simulink model "OMAP_ver_MIL10"  (R2018b)
settings: Solver=FixedStepDiscrete  StartTime=0.0  StopTime=10.0  FixedStep=0.01  RelTol=1e-3
undefined symbols (not defined in the file or in its folder): OMAP_Switch_EMS, OMAP_Switch_EPS, OMAP_Switch_ESC, OMAP_Switch_IC, OMAP_Switch_OTHER, TH_HMIClb_tiDgrdIconWarnHiDurT_C, TH_HMIClb_tiDgrdIconWarnLoDurT_C, TH_HMIClb_tiDgrdVocWarnDurT_C, TH_HMIClb_tiHndOffTxtWarnT_C, TH_HMIClb_tiHndOffVocWarnT_C, TH_HMIClb_tiSWALimFlgDetT_C, TH_HMIClb_tiTxtLimT_C
libraries: simulink x118
(part 3 of 9)

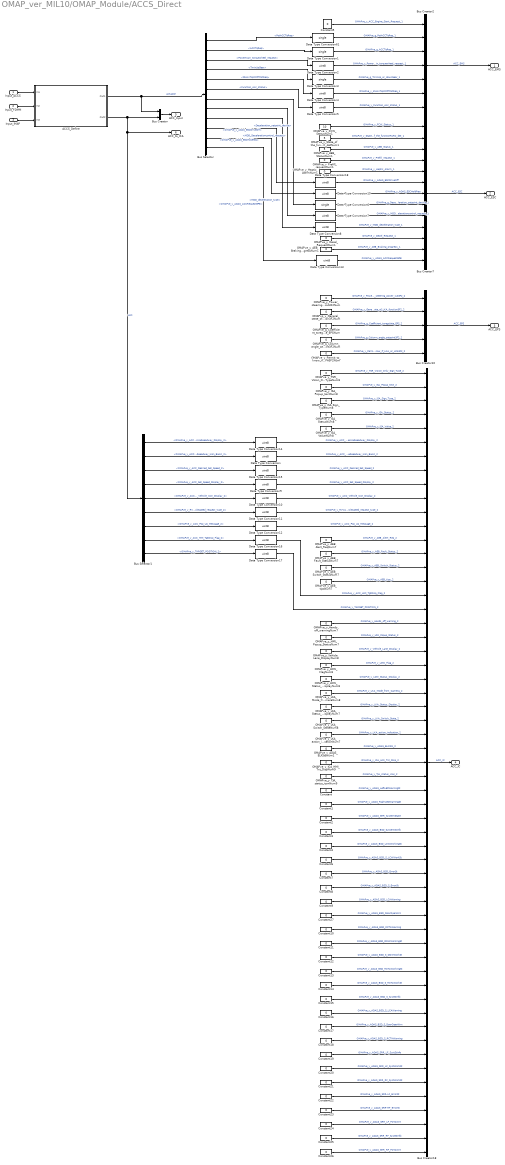
== system OMAP_ver_MIL10/OMAP_Module/ACCS_Direct ==
  Input_ACCS : Inport
  Input_FDMM : Inport  Port=2
  Input_IMAP : Inport  Port=3
  ACCS_Define : Subsystem
  Bus Creator : BusCreator  Inputs=2
  Bus Creator10 : BusCreator  Inputs=5
  Bus Creator18 : BusCreator  Inputs=57
  Bus Creator2 : BusCreator  Inputs=7
  Bus Creator7 : BusCreator  Inputs=13
  Bus Selector : BusSelector  OutputSignals=PotACCTqReq,ACCTqReq,Powertrain_torquewheel_request,TminUpGear,StAcvTqWhlPTPotReq,Function_Acc_status,Deceleration_setpoint_device,MDD_Decelerationcontrol_request,MDD_deceleration_type,OMAPve_y_ADAS_ESCDriveOff,OMAPve_y_ADAS_ESCHoldReq,OMAPve_y_ADAS_ACCRequestEPB
  Bus Selector1 : BusSelector  OutputSignals=OMAPve_y_ACC_DesiredHeadway_Display_2,OMAPve_y_ACC_DesiredHeadway_Icon_Basic_2,OMAPve_y_ACC_Desired_Set_Speed_2,OMAPve_y_ACC_Set_Speed_Display_2,OMAPve_y_ACC_Vehicle_Icon_Display_2,OMAPve_y_RVVACC_Vehiclespeed_request_type_2,OMAPve_y_ACC_Pop_Up_Message_2,OMAPve_y_ACC_HMI_TgtDisp_Flag_2,OMAPve_y_TARGET_POSITION_2
  Constant{,1..27} (28 alike) : Constant  Value=0  OutDataTypeStr=uint8
  Data Type Conversion{,2,4..5,7..19} (17 alike) : DataTypeConversion  OutDataTypeStr=uint8
  Data Type Conversion{1,3,6,61} (4 alike) : DataTypeConversion  OutDataTypeStr=single
  OMAPve_g_Coefficient_toregulate_EPSNum : Constant  Value=0  OutDataTypeStr=single
  OMAPve_g_Column_angle_setpoint3F2Num : Constant  Value=0  OutDataTypeStr=single
  OMAPve_y_ADAS_ELKStsNum1 : Constant  Value=0  OutDataTypeStr=uint8
  OMAPve_y_AEB_Alert_ReqNum7 : Constant  Value=0  OutDataTypeStr=uint8
  OMAPve_y_AEB_Braking_progressNum1 : Constant  Value=0  OutDataTypeStr=uint8
  OMAPve_y_AEB_Fault_StatusNum7 : Constant  Value=0  OutDataTypeStr=uint8
  OMAPve_y_AEB_StatusNum1 : Constant  Value=5  OutDataTypeStr=uint8
  OMAPve_y_AEB_Switch_StatusNum7 : Constant  Value=0  OutDataTypeStr=uint8
  OMAPve_y_AEB_tipsNum7 : Constant  Value=0  OutDataTypeStr=uint8
  OMAPve_y_Decel_RequestNum1 : Constant  Value=0  OutDataTypeStr=uint8
  OMAPve_y_FCW_StatusNum1 : Constant  Value=10  OutDataTypeStr=uint8
  OMAPve_y_General_state_of_LKA_function3F2Num : Constant  Value=0  OutDataTypeStr=uint8
  OMAPve_y_HMI_Popup_StatusNum7 : Constant  Value=0  OutDataTypeStr=uint8
  OMAPve_y_Hands_off_warningNum7 : Constant  Value=0  OutDataTypeStr=uint8
  OMAPve_y_Haptic_AlarmNum1 : Constant  Value=0  OutDataTypeStr=uint8
  OMAPve_y_ICA_HMI_Txt_DispNum9 : Constant  Value=0  OutDataTypeStr=uint8
  OMAPve_y_ISA_Popup_textNum8 : Constant  Value=0  OutDataTypeStr=uint8
  OMAPve_y_ISA_Sign_TypeNum8 : Constant  Value=0  OutDataTypeStr=uint8
  OMAPve_y_ISA_StatusNum8 : Constant  Value=0  OutDataTypeStr=uint8
  OMAPve_y_ISA_ValueNum8 : Constant  Value=0  OutDataTypeStr=uint8
  OMAPve_y_LDW_FlagNum8 : Constant  Value=0  OutDataTypeStr=uint8
  OMAPve_y_LDW_Status_DisplayNum8 : Constant  Value=0  OutDataTypeStr=uint8
  OMAPve_y_LKA_Mode_from_CameraNum8 : Constant  Value=0  OutDataTypeStr=uint8
  OMAPve_y_LKA_Status_DisplayNum7 : Constant  Value=0  OutDataTypeStr=uint8
  OMAPve_y_LKA_Switch_StateNum8 : Constant  Value=0  OutDataTypeStr=uint8
  OMAPve_y_LKA_action_indicationNum7 : Constant  Value=0  OutDataTypeStr=uint8
  OMAPve_y_Permit_to_know_if_LKA_or_LPA3F2Num : Constant  Value=0  OutDataTypeStr=uint8
  OMAPve_y_Power_steering_power_cut3F2Num : Constant  Value=0  OutDataTypeStr=uint8
  OMAPve_y_Prefill_requestNum1 : Constant  Value=0  OutDataTypeStr=uint8
  OMAPve_y_State_of_the_functionFARC_detNum1 : Constant  Value=5  OutDataTypeStr=uint8
  OMAPve_y_TJA_status_iconNum9 : Constant  Value=0  OutDataTypeStr=uint8
  OMAPve_y_TSR_Vision_Only_Sign_TypeNum8 : Constant  Value=0  OutDataTypeStr=uint8
  OMAPve_y_Vehicle_Lane_DisplayNum8 : Constant  Value=0  OutDataTypeStr=uint8
  ACC_EMS : Outport
  ACC_ESC : Outport  Port=2
  ACC_EPS : Outport  Port=3
  ACC_IC : Outport  Port=4
  ACC_Input : Outport  Port=5
  ACC_to_ICA : Outport  Port=6
  wires:
  Bus Selector/9 -> Data Type Conversion8/1  "<MDD_deceleration_type>"
  Bus Selector/8 -> Data Type Conversion7/1  "<MDD_Decelerationcontrol_request>"
  Bus Selector/7 -> Data Type Conversion6/1  "<Deceleration_setpoint_device>"
  Bus Selector/6 -> Data Type Conversion5/1  "<Function_Acc_status>"
  Bus Selector/5 -> Data Type Conversion4/1  "<StAcvTqWhlPTPotReq>"
  Bus Selector/4 -> Data Type Conversion3/1  "<TminUpGear>"
  Bus Selector/3 -> Data Type Conversion2/1  "<Powertrain_torquewheel_request>"
  Bus Selector/2 -> Data Type Conversion1/1  "<ACCTqReq>"
  Bus Selector/1 -> Data Type Conversion61/1  "<PotACCTqReq>"
  Input_FDMM/1 -> ACCS_Define/2(In2)
  Input_ACCS/1 -> ACCS_Define/1(In1)
  Bus Selector1/6 -> Data Type Conversion11/1  "<OMAPve_y_RVVACC_Vehiclespeed_request_type_2>"
  Bus Selector1/7 -> Data Type Conversion12/1  "<OMAPve_y_ACC_Pop_Up_Message_2>"
  Data Type Conversion1/1 -> Bus Creator2/3  "OMAPve_g_ACCTqReq_1"
  OMAPve_y_AEB_StatusNum1/1 -> Bus Creator7/3  "OMAPve_y_AEB_Status_1"
  Data Type Conversion6/1 -> Bus Creator7/8  "OMAPve_g_Deceleration_setpoint_device_1"
  Data Type Conversion8/1 -> Bus Creator7/10  "OMAPve_y_MDD_deceleration_type_1"
  Bus Selector1/5 -> Data Type Conversion10/1  "<OMAPve_y_ACC_Vehicle_Icon_Display_2>"
  Bus Creator18/1 -> ACC_IC/1  "ACC_IC"
  OMAPve_y_LDW_Status_DisplayNum8/1 -> Bus Creator18/23  "OMAPve_y_LDW_Status_Display_2"
  Bus Creator7/1 -> ACC_ESC/1  "ACC_ESC"
  OMAPve_y_AEB_tipsNum7/1 -> Bus Creator18/16  "OMAPve_y_AEB_tips_2"
  Bus Selector1/9 -> Data Type Conversion17/1  "<OMAPve_y_TARGET_POSITION_2>"
  Bus Selector1/3 -> Data Type Conversion15/1  "<OMAPve_y_ACC_Desired_Set_Speed_2>"
  Bus Selector1/1 -> Data Type Conversion14/1  "<OMAPve_y_ACC_DesiredHeadway_Display_2>"
  OMAPve_y_ISA_Sign_TypeNum8/1 -> Bus Creator18/3  "OMAPve_y_ISA_Sign_Type_2"
  OMAPve_y_HMI_Popup_StatusNum7/1 -> Bus Creator18/20  "OMAPve_y_HMI_Popup_Status_2"
  OMAPve_y_AEB_Alert_ReqNum7/1 -> Bus Creator18/13  "OMAPve_y_AEB_Alert_Req_2"
  Bus Creator2/1 -> ACC_EMS/1  "ACC_EMS"
  OMAPve_y_TSR_Vision_Only_Sign_TypeNum8/1 -> Bus Creator18/1  "OMAPve_y_TSR_Vision_Only_Sign_Type_2"
  OMAPve_y_LDW_FlagNum8/1 -> Bus Creator18/22  "OMAPve_y_LDW_Flag_2"
  OMAPve_y_AEB_Fault_StatusNum7/1 -> Bus Creator18/14  "OMAPve_y_AEB_Fault_Status_2"
  OMAPve_y_State_of_the_functionFARC_detNum1/1 -> Bus Creator7/2  "OMAPve_y_State_of_the_functionFARC_det_1"
  OMAPve_y_ISA_Popup_textNum8/1 -> Bus Creator18/2  "OMAPve_y_ISA_Popup_text_2"
  OMAPve_y_Haptic_AlarmNum1/1 -> Bus Creator7/5  "OMAPve_y_Haptic_Alarm_1"
  OMAPve_y_ICA_HMI_Txt_DispNum9/1 -> Bus Creator18/29  "OMAPve_y_ICA_HMI_Txt_Disp_2"
  Data Type Conversion4/1 -> Bus Creator2/6  "OMAPve_y_stAcvTqWhlPTPotReq_1"
  OMAPve_y_Decel_RequestNum1/1 -> Bus Creator7/11  "OMAPve_y_Decel_Request_1"
  Bus Selector1/2 -> Data Type Conversion/1  "<OMAPve_y_ACC_DesiredHeadway_Icon_Basic_2>"
  Data Type Conversion61/1 -> Bus Creator2/2  "OMAPve_g_PotACCTqReq_1"
  Bus Selector1/8 -> Data Type Conversion16/1  "<OMAPve_y_ACC_HMI_TgtDisp_Flag_2>"
  OMAPve_y_FCW_StatusNum1/1 -> Bus Creator7/1  "OMAPve_y_FCW_Status_1"
  OMAPve_y_Hands_off_warningNum7/1 -> Bus Creator18/19  "OMAPve_y_Hands_off_warning_2"
  OMAPve_y_ISA_ValueNum8/1 -> Bus Creator18/5  "OMAPve_y_ISA_Value_2"
  OMAPve_y_AEB_Braking_progressNum1/1 -> Bus Creator7/12  "OMAPve_y_AEB_Braking_progress_1"
  Data Type Conversion5/1 -> Bus Creator2/7  "OMAPve_y_Function_Acc_status_1"
  OMAPve_y_LKA_Status_DisplayNum7/1 -> Bus Creator18/25  "OMAPve_y_LKA_Status_Display_2"
  Data Type Conversion3/1 -> Bus Creator2/5  "OMAPve_g_TminUp_or_downGear_1"
  OMAPve_y_Vehicle_Lane_DisplayNum8/1 -> Bus Creator18/21  "OMAPve_y_Vehicle_Lane_Display_2"
  OMAPve_y_AEB_Switch_StatusNum7/1 -> Bus Creator18/15  "OMAPve_y_AEB_Switch_Status_2"
  Constant5/1 -> Bus Creator2/1  "OMAPve_y_ACC_Engine_Start_Request_1"
  OMAPve_y_TJA_status_iconNum9/1 -> Bus Creator18/30  "OMAPve_y_TJA_status_icon_2"
  OMAPve_y_LKA_action_indicationNum7/1 -> Bus Creator18/27  "OMAPve_y_LKA_action_indication_2"
  OMAPve_y_ISA_StatusNum8/1 -> Bus Creator18/4  "OMAPve_y_ISA_Status_2"
  Bus Selector1/4 -> Data Type Conversion9/1  "<OMAPve_y_ACC_Set_Speed_Display_2>"
  OMAPve_y_Prefill_requestNum1/1 -> Bus Creator7/4  "OMAPve_y_Prefill_request_1"
  Data Type Conversion7/1 -> Bus Creator7/9  "OMAPve_y_MDD_Decelerationcontrol_request_1"
  OMAPve_y_LKA_Switch_StateNum8/1 -> Bus Creator18/26  "OMAPve_y_LKA_Switch_State_2"
  Data Type Conversion2/1 -> Bus Creator2/4  "OMAPve_y_Powertrain_torquewheel_request_1"
  OMAPve_y_LKA_Mode_from_CameraNum8/1 -> Bus Creator18/24  "OMAPve_y_LKA_Mode_from_Camera_2"
  ACCS_Define/1(Out1) -> Bus Creator/1, Bus Selector/1  "actuator"
  OMAPve_y_Power_steering_power_cut3F2Num/1 -> Bus Creator10/1  "OMAPve_y_Power_steering_power_cut3F2_2"
  OMAPve_g_Coefficient_toregulate_EPSNum/1 -> Bus Creator10/3  "OMAPve_g_Coefficient_toregulate_EPS_2"
  OMAPve_y_Permit_to_know_if_LKA_or_LPA3F2Num/1 -> Bus Creator10/5  "OMAPve_y_Permit_to_know_if_LKA_or_LPA3F2_2"
  Bus Creator10/1 -> ACC_EPS/1  "ACC_EPS"
  OMAPve_y_General_state_of_LKA_function3F2Num/1 -> Bus Creator10/2  "OMAPve_y_General_state_of_LKA_function3F2_2"
  OMAPve_g_Column_angle_setpoint3F2Num/1 -> Bus Creator10/4  "OMAPve_g_Column_angle_setpoint3F2_2"
  Input_IMAP/1 -> ACCS_Define/3(In3)
  ACCS_Define/2(Out2) -> ACC_to_ICA/1, Bus Selector1/1, Bus Creator/2  "HMI"
  Bus Creator/1 -> ACC_Input/1
  Data Type Conversion/1 -> Bus Creator18/7  "OMAPve_y_ACC_DesiredHeadway_Icon_Basic_2"
  Data Type Conversion9/1 -> Bus Creator18/9  "OMAPve_y_ACC_Set_Speed_Display_2"
  Data Type Conversion10/1 -> Bus Creator18/10  "OMAPve_y_ACC_Vehicle_Icon_Display_2"
  Data Type Conversion11/1 -> Bus Creator18/11  "OMAPve_y_RVVACC_Vehiclespeed_request_type_2"
  Data Type Conversion12/1 -> Bus Creator18/12  "OMAPve_y_ACC_Pop_Up_Message_2"
  Data Type Conversion14/1 -> Bus Creator18/6  "OMAPve_y_ACC_DesiredHeadway_Display_2"
  Data Type Conversion15/1 -> Bus Creator18/8  "OMAPve_y_ACC_Desired_Set_Speed_2"
  Data Type Conversion16/1 -> Bus Creator18/17  "OMAPve_y_ACC_HMI_TgtDisp_Flag_2"
  Data Type Conversion17/1 -> Bus Creator18/18  "OMAPve_y_TARGET_POSITION_2"
  OMAPve_y_ADAS_ELKStsNum1/1 -> Bus Creator18/28  "OMAPve_y_ADAS_ELKSts_2"
  Data Type Conversion19/1 -> Bus Creator7/7  "OMAPve_y_ADAS_ESCHoldReq"
  Data Type Conversion18/1 -> Bus Creator7/6  "OMAPve_y_ADAS_ESCDriveOff"
  Bus Selector/10 -> Data Type Conversion18/1  "<OMAPve_y_ADAS_ESCDriveOff>"
  Bus Selector/11 -> Data Type Conversion19/1  "<OMAPve_y_ADAS_ESCHoldReq>"
  Data Type Conversion13/1 -> Bus Creator7/13  "OMAPve_y_ADAS_ACCRequestEPB"
  Bus Selector/12 -> Data Type Conversion13/1  "<OMAPve_y_ADAS_ACCRequestEPB>"
  Constant17/1 -> Bus Creator18/48  "OMAPve_y_ADAS_BSD_S_DoorOpenWrn"
  Constant16/1 -> Bus Creator18/47  "OMAPve_y_ADAS_BSD_S_LCAWarning"
  Constant1/1 -> Bus Creator18/32  "OMAPve_y_ADAS_RighrLEDWarningSt"
  Constant19/1 -> Bus Creator18/50  "OMAPve_y_ADAS_SRR_LF_SystStInfo"
  Constant10/1 -> Bus Creator18/41  "OMAPve_y_ADAS_BSD_RCTAWarning"
  Constant27/1 -> Bus Creator18/40  "OMAPve_y_ADAS_BSD_DoorOpenWrn"
  Constant22/1 -> Bus Creator18/53  "OMAPve_y_ADAS_SRR-LF_ErrorSt"
  Constant18/1 -> Bus Creator18/49  "OMAPve_y_ADAS_BSD_S_RCTAWarning"
  Constant20/1 -> Bus Creator18/51  "OMAPve_y_ADAS_SRR_LF_SystWorkSt"
  Constant21/1 -> Bus Creator18/52  "OMAPve_y_ADAS_SRR_RF_SystWorkSt"
  Constant15/1 -> Bus Creator18/46  "OMAPve_y_ADAS_BSD_S_SystStInfo"
  Constant14/1 -> Bus Creator18/45  "OMAPve_y_ADAS_BSD_S_RCTAWorkSt"
  Constant13/1 -> Bus Creator18/44  "OMAPve_y_ADAS_BSD_RCTAWorkingSt"
  Constant23/1 -> Bus Creator18/54  "OMAPve_y_ADAS_SRR-RF_ErrorSt"
  Constant26/1 -> Bus Creator18/57  "OMAPve_y_ADAS_SRR_RF_FCTAWrn"
  Constant/1 -> Bus Creator18/31  "OMAPve_y_ADAS_LeftLEDWarningSt"
  Constant25/1 -> Bus Creator18/56  "OMAPve_y_ADAS_SRR_RF_SystStInfo"
  Constant24/1 -> Bus Creator18/55  "OMAPve_y_ADAS_SRR_LF_FCTAWrn"
  Constant4/1 -> Bus Creator18/35  "OMAPve_y_ADAS_BSD_LCWWorkingSt"
  Constant9/1 -> Bus Creator18/39  "OMAPve_y_ADAS_BSD_LCAWarning"
  Constant12/1 -> Bus Creator18/43  "OMAPve_y_ADAS_BSD_S_DOWWorkSt"
  Constant6/1 -> Bus Creator18/36  "OMAPve_y_ADAS_BSD_S_LCWWorkSt"
  Constant8/1 -> Bus Creator18/38  "OMAPve_y_ADAS_BSD_S_ErrorSt"
  Constant2/1 -> Bus Creator18/33  "OMAPve_y_ADAS_SRR_SystemState"
  Constant7/1 -> Bus Creator18/37  "OMAPve_y_ADAS_BSD_ErrorSt"
  Constant3/1 -> Bus Creator18/34  "OMAPve_y_ADAS_BSD_SystemStInfo"
  Constant11/1 -> Bus Creator18/42  "OMAPve_y_ADAS_BSD_DOWWorkingSt"

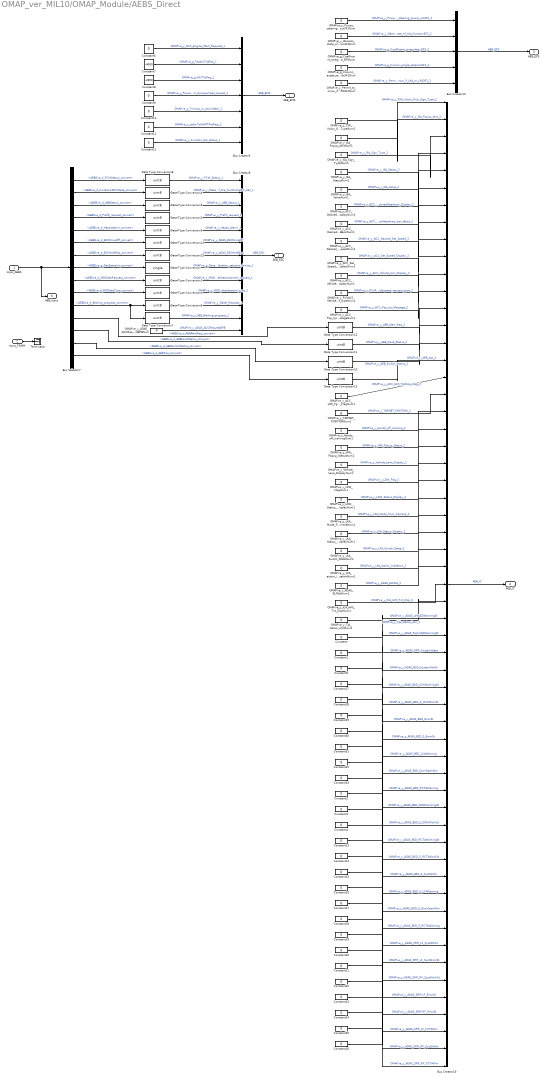
== system OMAP_ver_MIL10/OMAP_Module/AEBS_Direct ==
  Input_AEBS : Inport
  Input_FDMM : Inport  Port=2
  Bus Creator10 : BusCreator  Inputs=5
  Bus Creator19 : BusCreator  Inputs=57
  Bus Creator3 : BusCreator  Inputs=7
  Bus Creator8 : BusCreator  Inputs=13
  Bus Selector7 : BusSelector  OutputSignals=AEBSve_d_FCWStatus_convert,AEBSve_d_functionFARCState_convert,AEBSve_d_AEBStatus_convert,AEBSve_d_Prefill_request_convert,AEBSve_d_HapticAlarm_convert,AEBSve_d_ESCDriveOff_convert,AEBSve_d_ESCHoldReq_convert,AEBSve_g_DecSetpoint_convert,AEBSve_d_MDDdecRequest_convert,AEBSve_d_MDDdecType_convert,AEBSve_d_Braking_progress_convert,AEBSve_d_AEBAlertReq_convert,AEBSve_d_AEBFaultStatus_convert,AEBSve_d_AEBSwitchStatus_convert,AEBSve_d_AEBTips_convert
  Constant{,1..6,9,13..33} (29 alike) : Constant  Value=0  OutDataTypeStr=uint8
  Constant10 : Constant  Value=0  OutDataTypeStr=single
  Constant11 : Constant  Value=2  OutDataTypeStr=uint8
  Constant12 : Constant  Value=3  OutDataTypeStr=uint8
  Constant7 : Constant  Value=-4000  OutDataTypeStr=single
  Constant8 : Constant  Value=-4000  OutDataTypeStr=single
  Data Type Conversion : DataTypeConversion  OutDataTypeStr=single
  Data Type Conversion{1..15} (15 alike) : DataTypeConversion  OutDataTypeStr=uint8
  OMAPve_g_Coefficient_toregulate_EPSNum : Constant  Value=0  OutDataTypeStr=single
  OMAPve_g_Column_angle_setpoint3F2Num : Constant  Value=0  OutDataTypeStr=single
  OMAPve_y_ACC_DesiredHeadway_DisplayNum1 : Constant  Value=0  OutDataTypeStr=uint8
  OMAPve_y_ACC_DesiredHeadway_Icon_BasicNum1 : Constant  Value=0  OutDataTypeStr=uint8
  OMAPve_y_ACC_Desired_Set_SpeedNum1 : Constant  Value=0  OutDataTypeStr=uint8
  OMAPve_y_ACC_HMI_TgtDisp_FlagNum1 : Constant  Value=0  OutDataTypeStr=uint8
  OMAPve_y_ACC_Pop_Up_MessageNum1 : Constant  Value=0  OutDataTypeStr=uint8
  OMAPve_y_ACC_Set_Speed_DisplayNum1 : Constant  Value=0  OutDataTypeStr=uint8
  OMAPve_y_ACC_Vehicle_Icon_DisplayNum1 : Constant  Value=0  OutDataTypeStr=uint8
  OMAPve_y_ADAS_ACCRequestEPBNum : Constant  Value=0  OutDataTypeStr=uint8
  OMAPve_y_ADAS_ELKStsNum1 : Constant  Value=0  OutDataTypeStr=uint8
  OMAPve_y_General_state_of_LKA_function3F2Num : Constant  Value=0  OutDataTypeStr=uint8
  OMAPve_y_HMI_Popup_StatusNum1 : Constant  Value=0  OutDataTypeStr=uint8
  OMAPve_y_Hands_off_warningNum1 : Constant  Value=0  OutDataTypeStr=uint8
  OMAPve_y_ICA_HMI_Txt_DispNum1 : Constant  Value=0  OutDataTypeStr=uint8
  OMAPve_y_ISA_Popup_textNum1 : Constant  Value=0  OutDataTypeStr=uint8
  OMAPve_y_ISA_Sign_TypeNum1 : Constant  Value=0  OutDataTypeStr=uint8
  OMAPve_y_ISA_StatusNum1 : Constant  Value=0  OutDataTypeStr=uint8
  OMAPve_y_ISA_ValueNum1 : Constant  Value=0  OutDataTypeStr=uint8
  OMAPve_y_LDW_FlagNum1 : Constant  Value=0  OutDataTypeStr=uint8
  OMAPve_y_LDW_Status_DisplayNum1 : Constant  Value=0  OutDataTypeStr=uint8
  OMAPve_y_LKA_Mode_from_CameraNum1 : Constant  Value=0  OutDataTypeStr=uint8
  OMAPve_y_LKA_Status_DisplayNum1 : Constant  Value=0  OutDataTypeStr=uint8
  OMAPve_y_LKA_Switch_StateNum1 : Constant  Value=0  OutDataTypeStr=uint8
  OMAPve_y_LKA_action_indicationNum1 : Constant  Value=0  OutDataTypeStr=uint8
  OMAPve_y_Permit_to_know_if_LKA_or_LPA3F2Num : Constant  Value=0  OutDataTypeStr=uint8
  OMAPve_y_Power_steering_power_cut3F2Num : Constant  Value=0  OutDataTypeStr=uint8
  OMAPve_y_RVVACC_Vehiclespeed_request_typeNum1 : Constant  Value=0  OutDataTypeStr=uint8
  OMAPve_y_TARGET_POSITIONNum1 : Constant  Value=6  OutDataTypeStr=uint8
  OMAPve_y_TJA_status_iconNum1 : Constant  Value=0  OutDataTypeStr=uint8
  OMAPve_y_TSR_Vision_Only_Sign_TypeNum1 : Constant  Value=0  OutDataTypeStr=uint8
  OMAPve_y_Vehicle_Lane_DisplayNum1 : Constant  Value=0  OutDataTypeStr=uint8
  Terminator : Terminator
  AEB_EMS : Outport
  AEB_ESC : Outport  Port=2
  AEB_EPS : Outport  Port=3
  AEB_IC : Outport  Port=4
  AEB_Input : Outport  Port=5
  wires:
  OMAPve_y_LDW_FlagNum1/1 -> Bus Creator19/22  "OMAPve_y_LDW_Flag_2"
  Bus Selector7/15 -> Data Type Conversion13/1  "<AEBSve_d_AEBTips_convert>"
  OMAPve_y_Vehicle_Lane_DisplayNum1/1 -> Bus Creator19/21  "OMAPve_y_Vehicle_Lane_Display_2"
  Bus Selector7/1 -> Data Type Conversion8/1  "<AEBSve_d_FCWStatus_convert>"
  OMAPve_y_ISA_ValueNum1/1 -> Bus Creator19/5  "OMAPve_y_ISA_Value_2"
  Bus Selector7/8 -> Data Type Conversion/1  "<AEBSve_g_DecSetpoint_convert>"
  OMAPve_y_ACC_DesiredHeadway_DisplayNum1/1 -> Bus Creator19/6  "OMAPve_y_ACC_DesiredHeadway_Display_2"
  Data Type Conversion13/1 -> Bus Creator19/16  "OMAPve_y_AEB_tips_2"
  OMAPve_y_HMI_Popup_StatusNum1/1 -> Bus Creator19/20  "OMAPve_y_HMI_Popup_Status_2"
  OMAPve_y_Hands_off_warningNum1/1 -> Bus Creator19/19  "OMAPve_y_Hands_off_warning_2"
  Bus Creator3/1 -> AEB_EMS/1  "AEB_EMS"
  OMAPve_y_ACC_DesiredHeadway_Icon_BasicNum1/1 -> Bus Creator19/7  "OMAPve_y_ACC_DesiredHeadway_Icon_Basic_2"
  Constant9/1 -> Bus Creator3/4  "OMAPve_y_Powertrain_torquewheel_request_1"
  OMAPve_y_ACC_Vehicle_Icon_DisplayNum1/1 -> Bus Creator19/10  "OMAPve_y_ACC_Vehicle_Icon_Display_2"
  OMAPve_y_ISA_Sign_TypeNum1/1 -> Bus Creator19/3  "OMAPve_y_ISA_Sign_Type_2"
  Data Type Conversion9/1 -> Bus Creator8/5  "OMAPve_y_Haptic_Alarm_1"
  Data Type Conversion2/1 -> Bus Creator8/4  "OMAPve_y_Prefill_request_1"
  Bus Selector7/13 -> Data Type Conversion11/1  "<AEBSve_d_AEBFaultStatus_convert>"
  OMAPve_y_LKA_Switch_StateNum1/1 -> Bus Creator19/26  "OMAPve_y_LKA_Switch_State_2"
  OMAPve_y_ISA_Popup_textNum1/1 -> Bus Creator19/2  "OMAPve_y_ISA_Popup_text_2"
  Bus Selector7/3 -> Data Type Conversion5/1  "<AEBSve_d_AEBStatus_convert>"
  Bus Selector7/2 -> Data Type Conversion4/1  "<AEBSve_d_functionFARCState_convert>"
  Data Type Conversion10/1 -> Bus Creator19/15  "OMAPve_y_AEB_Switch_Status_2"
  OMAPve_y_TARGET_POSITIONNum1/1 -> Bus Creator19/18  "OMAPve_y_TARGET_POSITION_2"
  Bus Selector7/4 -> Data Type Conversion2/1  "<AEBSve_d_Prefill_request_convert>"
  OMAPve_y_RVVACC_Vehiclespeed_request_typeNum1/1 -> Bus Creator19/11  "OMAPve_y_RVVACC_Vehiclespeed_request_type_2"
  Input_AEBS/1 -> AEB_Input/1, Bus Selector7/1
  Bus Selector7/12 -> Data Type Conversion12/1  "<AEBSve_d_AEBAlertReq_convert>"
  Bus Creator19/1 -> AEB_IC/1  "AEB_IC"
  Bus Creator8/1 -> AEB_ESC/1  "AEB_ESC"
  OMAPve_y_LDW_Status_DisplayNum1/1 -> Bus Creator19/23  "OMAPve_y_LDW_Status_Display_2"
  Bus Selector7/10 -> Data Type Conversion3/1  "<AEBSve_d_MDDdecType_convert>"
  OMAPve_y_ACC_Set_Speed_DisplayNum1/1 -> Bus Creator19/9  "OMAPve_y_ACC_Set_Speed_Display_2"
  OMAPve_y_LKA_Mode_from_CameraNum1/1 -> Bus Creator19/24  "OMAPve_y_LKA_Mode_from_Camera_2"
  Bus Selector7/14 -> Data Type Conversion10/1  "<AEBSve_d_AEBSwitchStatus_convert>"
  Data Type Conversion12/1 -> Bus Creator19/13  "OMAPve_y_AEB_Alert_Req_2"
  OMAPve_y_ACC_Desired_Set_SpeedNum1/1 -> Bus Creator19/8  "OMAPve_y_ACC_Desired_Set_Speed_2"
  Data Type Conversion7/1 -> Bus Creator8/12  "OMAPve_y_AEB_Braking_progress_1"
  Data Type Conversion11/1 -> Bus Creator19/14  "OMAPve_y_AEB_Fault_Status_2"
  OMAPve_y_ICA_HMI_Txt_DispNum1/1 -> Bus Creator19/29  "OMAPve_y_ICA_HMI_Txt_Disp_2"
  OMAPve_y_ACC_Pop_Up_MessageNum1/1 -> Bus Creator19/12  "OMAPve_y_ACC_Pop_Up_Message_2"
  Bus Selector7/11 -> Data Type Conversion7/1, Data Type Conversion6/1  "<AEBSve_d_Braking_progress_convert>"
  Data Type Conversion6/1 -> Bus Creator8/11  "OMAPve_y_Decel_Request_1"
  OMAPve_y_LKA_action_indicationNum1/1 -> Bus Creator19/27  "OMAPve_y_LKA_action_indication_2"
  Constant12/1 -> Bus Creator3/7  "OMAPve_y_Function_Acc_status_1"
  OMAPve_y_LKA_Status_DisplayNum1/1 -> Bus Creator19/25  "OMAPve_y_LKA_Status_Display_2"
  OMAPve_y_ISA_StatusNum1/1 -> Bus Creator19/4  "OMAPve_y_ISA_Status_2"
  Data Type Conversion4/1 -> Bus Creator8/2  "OMAPve_y_State_of_the_functionFARC_det_1"
  Data Type Conversion5/1 -> Bus Creator8/3  "OMAPve_y_AEB_Status_1"
  OMAPve_y_TJA_status_iconNum1/1 -> Bus Creator19/30  "OMAPve_y_TJA_status_icon_2"
  Data Type Conversion8/1 -> Bus Creator8/1  "OMAPve_y_FCW_Status_1"
  OMAPve_y_ACC_HMI_TgtDisp_FlagNum1/1 -> Bus Creator19/17  "OMAPve_y_ACC_HMI_TgtDisp_Flag_2"
  OMAPve_y_TSR_Vision_Only_Sign_TypeNum1/1 -> Bus Creator19/1  "OMAPve_y_TSR_Vision_Only_Sign_Type_2"
  Data Type Conversion3/1 -> Bus Creator8/10  "OMAPve_y_MDD_deceleration_type_1"
  Bus Selector7/5 -> Data Type Conversion9/1  "<AEBSve_d_HapticAlarm_convert>"
  Constant11/1 -> Bus Creator3/6  "OMAPve_y_stAcvTqWhlPTPotReq_1"
  Constant8/1 -> Bus Creator3/3  "OMAPve_g_ACCTqReq_1"
  Constant10/1 -> Bus Creator3/5  "OMAPve_g_TminUp_or_downGear_1"
  Constant6/1 -> Bus Creator3/1  "OMAPve_y_ACC_Engine_Start_Request_1"
  Constant7/1 -> Bus Creator3/2  "OMAPve_g_PotACCTqReq_1"
  Bus Selector7/9 -> Data Type Conversion1/1  "<AEBSve_d_MDDdecRequest_convert>"
  Data Type Conversion/1 -> Bus Creator8/8  "OMAPve_g_Deceleration_setpoint_device_1"
  Data Type Conversion1/1 -> Bus Creator8/9  "OMAPve_y_MDD_Decelerationcontrol_request_1"
  OMAPve_g_Coefficient_toregulate_EPSNum/1 -> Bus Creator10/3  "OMAPve_g_Coefficient_toregulate_EPS_2"
  OMAPve_y_Power_steering_power_cut3F2Num/1 -> Bus Creator10/1  "OMAPve_y_Power_steering_power_cut3F2_2"
  OMAPve_y_General_state_of_LKA_function3F2Num/1 -> Bus Creator10/2  "OMAPve_y_General_state_of_LKA_function3F2_2"
  Bus Creator10/1 -> AEB_EPS/1  "AEB_EPS"
  OMAPve_y_Permit_to_know_if_LKA_or_LPA3F2Num/1 -> Bus Creator10/5  "OMAPve_y_Permit_to_know_if_LKA_or_LPA3F2_2"
  OMAPve_g_Column_angle_setpoint3F2Num/1 -> Bus Creator10/4  "OMAPve_g_Column_angle_setpoint3F2_2"
  Input_FDMM/1 -> Terminator/1
  OMAPve_y_ADAS_ELKStsNum1/1 -> Bus Creator19/28  "OMAPve_y_ADAS_ELKSts_2"
  Data Type Conversion14/1 -> Bus Creator8/6  "OMAPve_y_ADAS_ESCDriveOff"
  Data Type Conversion15/1 -> Bus Creator8/7  "OMAPve_y_ADAS_ESCHoldReq"
  Bus Selector7/6 -> Data Type Conversion14/1  "<AEBSve_d_ESCDriveOff_convert>"
  Bus Selector7/7 -> Data Type Conversion15/1  "<AEBSve_d_ESCHoldReq_convert>"
  OMAPve_y_ADAS_ACCRequestEPBNum/1 -> Bus Creator8/13  "OMAPve_y_ADAS_ACCRequestEPB"
  Constant17/1 -> Bus Creator19/48  "OMAPve_y_ADAS_BSD_S_DoorOpenWrn"
  Constant16/1 -> Bus Creator19/47  "OMAPve_y_ADAS_BSD_S_LCAWarning"
  Constant1/1 -> Bus Creator19/32  "OMAPve_y_ADAS_RighrLEDWarningSt"
  Constant19/1 -> Bus Creator19/50  "OMAPve_y_ADAS_SRR_LF_SystStInfo"
  Constant2/1 -> Bus Creator19/41  "OMAPve_y_ADAS_BSD_RCTAWarning"
  Constant33/1 -> Bus Creator19/40  "OMAPve_y_ADAS_BSD_DoorOpenWrn"
  Constant22/1 -> Bus Creator19/53  "OMAPve_y_ADAS_SRR-LF_ErrorSt"
  Constant18/1 -> Bus Creator19/49  "OMAPve_y_ADAS_BSD_S_RCTAWarning"
  Constant20/1 -> Bus Creator19/51  "OMAPve_y_ADAS_SRR_LF_SystWorkSt"
  Constant21/1 -> Bus Creator19/52  "OMAPve_y_ADAS_SRR_RF_SystWorkSt"
  Constant15/1 -> Bus Creator19/46  "OMAPve_y_ADAS_BSD_S_SystStInfo"
  Constant14/1 -> Bus Creator19/45  "OMAPve_y_ADAS_BSD_S_RCTAWorkSt"
  Constant13/1 -> Bus Creator19/44  "OMAPve_y_ADAS_BSD_RCTAWorkingSt"
  Constant23/1 -> Bus Creator19/54  "OMAPve_y_ADAS_SRR-RF_ErrorSt"
  Constant26/1 -> Bus Creator19/57  "OMAPve_y_ADAS_SRR_RF_FCTAWrn"
  Constant/1 -> Bus Creator19/31  "OMAPve_y_ADAS_LeftLEDWarningSt"
  Constant25/1 -> Bus Creator19/56  "OMAPve_y_ADAS_SRR_RF_SystStInfo"
  Constant24/1 -> Bus Creator19/55  "OMAPve_y_ADAS_SRR_LF_FCTAWrn"
  Constant28/1 -> Bus Creator19/35  "OMAPve_y_ADAS_BSD_LCWWorkingSt"
  Constant32/1 -> Bus Creator19/39  "OMAPve_y_ADAS_BSD_LCAWarning"
  Constant4/1 -> Bus Creator19/43  "OMAPve_y_ADAS_BSD_S_DOWWorkSt"
  Constant29/1 -> Bus Creator19/36  "OMAPve_y_ADAS_BSD_S_LCWWorkSt"
  Constant31/1 -> Bus Creator19/38  "OMAPve_y_ADAS_BSD_S_ErrorSt"
  Constant5/1 -> Bus Creator19/33  "OMAPve_y_ADAS_SRR_SystemState"
  Constant30/1 -> Bus Creator19/37  "OMAPve_y_ADAS_BSD_ErrorSt"
  Constant27/1 -> Bus Creator19/34  "OMAPve_y_ADAS_BSD_SystemStInfo"
  Constant3/1 -> Bus Creator19/42  "OMAPve_y_ADAS_BSD_DOWWorkingSt"

== system OMAP_ver_MIL10/OMAP_Module/CHecksum_Rollingcounter ==
  OMAPve_y_CHKSUM_TRMENum : Constant  Value=0  OutDataTypeStr=uint8
  OMAPve_y_CHKSUM_TRME_1 : DataTypeConversion  OutDataTypeStr=UInt8
  OMAPve_y_CHKSUM_TRME_DYN_ACC2Num : Constant  Value=0  OutDataTypeStr=uint8
  OMAPve_y_CHKSUM_TRME_DYN_ACC2_1 : DataTypeConversion  OutDataTypeStr=UInt8
  OMAPve_y_CHKSUM_TRME_DYN_ACCNum : Constant  Value=0  OutDataTypeStr=uint8
  OMAPve_y_CHKSUM_TRME_DYN_ACC_1 : DataTypeConversion  OutDataTypeStr=UInt8
  OMAPve_y_CPT_PROCESSNum : Constant  Value=0  OutDataTypeStr=uint8
  OMAPve_y_CPT_PROCESS_1 : DataTypeConversion  OutDataTypeStr=UInt8
  OMAPve_y_CPT_PROCESS_4B_ACC2Num : Constant  Value=0  OutDataTypeStr=uint8
  OMAPve_y_CPT_PROCESS_4B_ACC2_1 : DataTypeConversion  OutDataTypeStr=UInt8
  OMAPve_y_CPT_PROCESS_4B_ACCNum : Constant  Value=0  OutDataTypeStr=uint8
  OMAPve_y_CPT_PROCESS_4B_ACC_1 : DataTypeConversion  OutDataTypeStr=UInt8
  Terminator{,1..5} (6 alike) : Terminator
  wires:
  OMAPve_y_CHKSUM_TRME_1/1 -> Terminator4/1
  OMAPve_y_CHKSUM_TRME_DYN_ACC2Num/1 -> OMAPve_y_CHKSUM_TRME_DYN_ACC2_1/1
  OMAPve_y_CHKSUM_TRME_DYN_ACCNum/1 -> OMAPve_y_CHKSUM_TRME_DYN_ACC_1/1
  OMAPve_y_CPT_PROCESS_4B_ACC_1/1 -> Terminator/1
  OMAPve_y_CHKSUM_TRMENum/1 -> OMAPve_y_CHKSUM_TRME_1/1
  OMAPve_y_CHKSUM_TRME_DYN_ACC_1/1 -> Terminator1/1
  OMAPve_y_CPT_PROCESS_1/1 -> Terminator5/1
  OMAPve_y_CHKSUM_TRME_DYN_ACC2_1/1 -> Terminator3/1
  OMAPve_y_CPT_PROCESS_4B_ACCNum/1 -> OMAPve_y_CPT_PROCESS_4B_ACC_1/1
  OMAPve_y_CPT_PROCESS_4B_ACC2_1/1 -> Terminator2/1
  OMAPve_y_CPT_PROCESS_4B_ACC2Num/1 -> OMAPve_y_CPT_PROCESS_4B_ACC2_1/1
  OMAPve_y_CPT_PROCESSNum/1 -> OMAPve_y_CPT_PROCESS_1/1

== system OMAP_ver_MIL10/OMAP_Module/Default_EMS ==
  Bus Creator : BusCreator  Inputs=7
  OMAPve_g_ACCTqReqNum : Constant  Value=-4000  OutDataTypeStr=single
  OMAPve_g_PotACCTqReqNum : Constant  Value=-4000  OutDataTypeStr=single
  OMAPve_g_TminUp_or_downGearNum : Constant  Value=6.2  OutDataTypeStr=single
  OMAPve_y_ACC_Engine_Start_RequestNum : Constant  Value=0  OutDataTypeStr=uint8
  OMAPve_y_Function_Acc_statusNum : Constant  Value=3  OutDataTypeStr=uint8
  OMAPve_y_Powertrain_torquewheel_requestNum : Constant  Value=0  OutDataTypeStr=uint8
  OMAPve_y_stAcvTqWhlPTPotReqNum : Constant  Value=0  OutDataTypeStr=uint8
  Default_EMS : Outport
  wires:
  OMAPve_y_ACC_Engine_Start_RequestNum/1 -> Bus Creator/1  "OMAPve_y_ACC_Engine_Start_Request_1"
  OMAPve_y_Function_Acc_statusNum/1 -> Bus Creator/7  "OMAPve_y_Function_Acc_status_1"
  OMAPve_y_stAcvTqWhlPTPotReqNum/1 -> Bus Creator/6  "OMAPve_y_stAcvTqWhlPTPotReq_1"
  OMAPve_y_Powertrain_torquewheel_requestNum/1 -> Bus Creator/4  "OMAPve_y_Powertrain_torquewheel_request_1"
  Bus Creator/1 -> Default_EMS/1  "Default_EMS"
  OMAPve_g_ACCTqReqNum/1 -> Bus Creator/3  "OMAPve_g_ACCTqReq_1"
  OMAPve_g_PotACCTqReqNum/1 -> Bus Creator/2  "OMAPve_g_PotACCTqReq_1"
  OMAPve_g_TminUp_or_downGearNum/1 -> Bus Creator/5  "OMAPve_g_TminUp_or_downGear_1"

== system OMAP_ver_MIL10/OMAP_Module/Default_EPS ==
  Bus Creator10 : BusCreator  Inputs=5
  OMAPve_g_Coefficient_toregulate_EPSNum : Constant  Value=0  OutDataTypeStr=single
  OMAPve_g_Column_angle_setpoint3F2Num : Constant  Value=0  OutDataTypeStr=single
  OMAPve_y_General_state_of_LKA_function3F2Num : Constant  Value=0  OutDataTypeStr=uint8
  OMAPve_y_Permit_to_know_if_LKA_or_LPA3F2Num : Constant  Value=0  OutDataTypeStr=uint8
  OMAPve_y_Power_steering_power_cut3F2Num : Constant  Value=0  OutDataTypeStr=uint8
  Default_EPS : Outport
  wires:
  OMAPve_y_Power_steering_power_cut3F2Num/1 -> Bus Creator10/1  "OMAPve_y_Power_steering_power_cut3F2_2"
  OMAPve_y_General_state_of_LKA_function3F2Num/1 -> Bus Creator10/2  "OMAPve_y_General_state_of_LKA_function3F2_2"
  Bus Creator10/1 -> Default_EPS/1  "Default_EPS"
  OMAPve_g_Coefficient_toregulate_EPSNum/1 -> Bus Creator10/3  "OMAPve_g_Coefficient_toregulate_EPS_2"
  OMAPve_y_Permit_to_know_if_LKA_or_LPA3F2Num/1 -> Bus Creator10/5  "OMAPve_y_Permit_to_know_if_LKA_or_LPA3F2_2"
  OMAPve_g_Column_angle_setpoint3F2Num/1 -> Bus Creator10/4  "OMAPve_g_Column_angle_setpoint3F2_2"

== system OMAP_ver_MIL10/OMAP_Module/Default_ESC ==
  Bus Creator5 : BusCreator  Inputs=13
  OMAPve_g_Deceleration_setpoint_deviceNum : Constant  Value=2.05  OutDataTypeStr=single
  OMAPve_y_ADAS_ACCRequestEPBNum : Constant  Value=0  OutDataTypeStr=uint8
  OMAPve_y_ADAS_ESCDriveOffNum : Constant  Value=0  OutDataTypeStr=uint8
  OMAPve_y_ADAS_ESCHoldReqNum : Constant  Value=0  OutDataTypeStr=uint8
  OMAPve_y_AEB_Braking_progressNum : Constant  Value=0  OutDataTypeStr=uint8
  OMAPve_y_AEB_StatusNum : Constant  Value=0  OutDataTypeStr=uint8
  OMAPve_y_Decel_RequestNum : Constant  Value=0  OutDataTypeStr=uint8
  OMAPve_y_FCW_StatusNum : Constant  Value=10  OutDataTypeStr=uint8
  OMAPve_y_Haptic_AlarmNum : Constant  Value=0  OutDataTypeStr=uint8
  OMAPve_y_MDD_Decelerationcontrol_requestNum : Constant  Value=0  OutDataTypeStr=uint8
  OMAPve_y_MDD_deceleration_typeNum : Constant  Value=0  OutDataTypeStr=uint8
  OMAPve_y_Prefill_requestNum : Constant  Value=0  OutDataTypeStr=uint8
  OMAPve_y_State_of_the_functionFARC_detNum : Constant  Value=0  OutDataTypeStr=uint8
  Default_ESC : Outport
  wires:
  OMAPve_g_Deceleration_setpoint_deviceNum/1 -> Bus Creator5/8  "OMAPve_g_Deceleration_setpoint_device_1"
  OMAPve_y_FCW_StatusNum/1 -> Bus Creator5/1  "OMAPve_y_FCW_Status_1"
  OMAPve_y_Haptic_AlarmNum/1 -> Bus Creator5/5  "OMAPve_y_Haptic_Alarm_1"
  OMAPve_y_State_of_the_functionFARC_detNum/1 -> Bus Creator5/2  "OMAPve_y_State_of_the_functionFARC_det_1"
  OMAPve_y_AEB_Braking_progressNum/1 -> Bus Creator5/12  "OMAPve_y_AEB_Braking_progress_1"
  OMAPve_y_Decel_RequestNum/1 -> Bus Creator5/11  "OMAPve_y_Decel_Request_1"
  OMAPve_y_MDD_deceleration_typeNum/1 -> Bus Creator5/10  "OMAPve_y_MDD_deceleration_type_1"
  OMAPve_y_AEB_StatusNum/1 -> Bus Creator5/3  "OMAPve_y_AEB_Status_1"
  Bus Creator5/1 -> Default_ESC/1  "Default_ESC"
  OMAPve_y_Prefill_requestNum/1 -> Bus Creator5/4  "OMAPve_y_Prefill_request_1"
  OMAPve_y_MDD_Decelerationcontrol_requestNum/1 -> Bus Creator5/9  "OMAPve_y_MDD_Decelerationcontrol_request_1"
  OMAPve_y_ADAS_ESCDriveOffNum/1 -> Bus Creator5/6  "OMAPve_y_ADAS_ESCDriveOff"
  OMAPve_y_ADAS_ESCHoldReqNum/1 -> Bus Creator5/7  "OMAPve_y_ADAS_ESCHoldReq"
  OMAPve_y_ADAS_ACCRequestEPBNum/1 -> Bus Creator5/13  "OMAPve_y_ADAS_ACCRequestEPB"

== system OMAP_ver_MIL10/OMAP_Module/Default_IC ==
  Bus Creator16 : BusCreator  Inputs=57
  Constant{,1..26} (27 alike) : Constant  Value=0  OutDataTypeStr=uint8
  OMAPve_y_ACC_DesiredHeadway_DisplayNum : Constant  Value=0  OutDataTypeStr=uint8
  OMAPve_y_ACC_DesiredHeadway_Icon_BasicNum : Constant  Value=0  OutDataTypeStr=uint8
  OMAPve_y_ACC_Desired_Set_SpeedNum : Constant  Value=0  OutDataTypeStr=uint8
  OMAPve_y_ACC_HMI_TgtDisp_FlagNum : Constant  Value=0  OutDataTypeStr=uint8
  OMAPve_y_ACC_Pop_Up_MessageNum : Constant  Value=0  OutDataTypeStr=uint8
  OMAPve_y_ACC_Set_Speed_DisplayNum : Constant  Value=0  OutDataTypeStr=uint8
  OMAPve_y_ACC_Vehicle_Icon_DisplayNum : Constant  Value=0  OutDataTypeStr=uint8
  OMAPve_y_ADAS_ELKStsNum1 : Constant  Value=0  OutDataTypeStr=uint8
  OMAPve_y_AEB_Alert_ReqNum : Constant  Value=0  OutDataTypeStr=uint8
  OMAPve_y_AEB_Fault_StatusNum : Constant  Value=0  OutDataTypeStr=uint8
  OMAPve_y_AEB_Switch_StatusNum : Constant  Value=0  OutDataTypeStr=uint8
  OMAPve_y_AEB_tipsNum : Constant  Value=0  OutDataTypeStr=uint8
  OMAPve_y_HMI_Popup_StatusNum : Constant  Value=0  OutDataTypeStr=uint8
  OMAPve_y_Hands_off_warningNum : Constant  Value=0  OutDataTypeStr=uint8
  OMAPve_y_ICA_HMI_Txt_DispNum : Constant  Value=0  OutDataTypeStr=uint8
  OMAPve_y_ISA_Popup_textNum : Constant  Value=0  OutDataTypeStr=uint8
  OMAPve_y_ISA_Sign_TypeNum : Constant  Value=0  OutDataTypeStr=uint8
  OMAPve_y_ISA_StatusNum : Constant  Value=0  OutDataTypeStr=uint8
  OMAPve_y_ISA_ValueNum : Constant  Value=0  OutDataTypeStr=uint8
  OMAPve_y_LDW_FlagNum : Constant  Value=0  OutDataTypeStr=uint8
  OMAPve_y_LDW_Status_DisplayNum : Constant  Value=0  OutDataTypeStr=uint8
  OMAPve_y_LKA_Mode_from_CameraNum : Constant  Value=0  OutDataTypeStr=uint8
  OMAPve_y_LKA_Status_DisplayNum : Constant  Value=0  OutDataTypeStr=uint8
  OMAPve_y_LKA_Switch_StateNum : Constant  Value=0  OutDataTypeStr=uint8
  OMAPve_y_LKA_action_indicationNum : Constant  Value=0  OutDataTypeStr=uint8
  OMAPve_y_RVVACC_Vehiclespeed_request_typeNum : Constant  Value=0  OutDataTypeStr=uint8
  OMAPve_y_TARGET_POSITIONNum : Constant  Value=6  OutDataTypeStr=uint8
  OMAPve_y_TJA_status_iconNum : Constant  Value=0  OutDataTypeStr=uint8
  OMAPve_y_TSR_Vision_Only_Sign_TypeNum : Constant  Value=0  OutDataTypeStr=uint8
  OMAPve_y_Vehicle_Lane_DisplayNum : Constant  Value=0  OutDataTypeStr=uint8
  Default_IC : Outport
  wires:
  OMAPve_y_LKA_Status_DisplayNum/1 -> Bus Creator16/25  "OMAPve_y_LKA_Status_Display_2"
  OMAPve_y_ACC_Desired_Set_SpeedNum/1 -> Bus Creator16/8  "OMAPve_y_ACC_Desired_Set_Speed_2"
  OMAPve_y_AEB_tipsNum/1 -> Bus Creator16/16  "OMAPve_y_AEB_tips_2"
  OMAPve_y_ACC_Pop_Up_MessageNum/1 -> Bus Creator16/12  "OMAPve_y_ACC_Pop_Up_Message_2"
  OMAPve_y_ISA_Sign_TypeNum/1 -> Bus Creator16/3  "OMAPve_y_ISA_Sign_Type_2"
  OMAPve_y_ISA_StatusNum/1 -> Bus Creator16/4  "OMAPve_y_ISA_Status_2"
  OMAPve_y_LDW_Status_DisplayNum/1 -> Bus Creator16/23  "OMAPve_y_LDW_Status_Display_2"
  OMAPve_y_AEB_Switch_StatusNum/1 -> Bus Creator16/15  "OMAPve_y_AEB_Switch_Status_2"
  OMAPve_y_ACC_DesiredHeadway_Icon_BasicNum/1 -> Bus Creator16/7  "OMAPve_y_ACC_DesiredHeadway_Icon_Basic_2"
  OMAPve_y_ICA_HMI_Txt_DispNum/1 -> Bus Creator16/29  "OMAPve_y_ICA_HMI_Txt_Disp_2"
  OMAPve_y_TARGET_POSITIONNum/1 -> Bus Creator16/18  "OMAPve_y_TARGET_POSITION_2"
  OMAPve_y_ISA_ValueNum/1 -> Bus Creator16/5  "OMAPve_y_ISA_Value_2"
  OMAPve_y_ACC_Vehicle_Icon_DisplayNum/1 -> Bus Creator16/10  "OMAPve_y_ACC_Vehicle_Icon_Display_2"
  OMAPve_y_ACC_DesiredHeadway_DisplayNum/1 -> Bus Creator16/6  "OMAPve_y_ACC_DesiredHeadway_Display_2"
  OMAPve_y_AEB_Alert_ReqNum/1 -> Bus Creator16/13  "OMAPve_y_AEB_Alert_Req_2"
  OMAPve_y_ISA_Popup_textNum/1 -> Bus Creator16/2  "OMAPve_y_ISA_Popup_text_2"
  OMAPve_y_ACC_Set_Speed_DisplayNum/1 -> Bus Creator16/9  "OMAPve_y_ACC_Set_Speed_Display_2"
  OMAPve_y_LKA_action_indicationNum/1 -> Bus Creator16/27  "OMAPve_y_LKA_action_indication_2"
  OMAPve_y_Hands_off_warningNum/1 -> Bus Creator16/19  "OMAPve_y_Hands_off_warning_2"
  OMAPve_y_RVVACC_Vehiclespeed_request_typeNum/1 -> Bus Creator16/11  "OMAPve_y_RVVACC_Vehiclespeed_request_type_2"
  OMAPve_y_LKA_Mode_from_CameraNum/1 -> Bus Creator16/24  "OMAPve_y_LKA_Mode_from_Camera_2"
  OMAPve_y_ACC_HMI_TgtDisp_FlagNum/1 -> Bus Creator16/17  "OMAPve_y_ACC_HMI_TgtDisp_Flag_2"
  OMAPve_y_HMI_Popup_StatusNum/1 -> Bus Creator16/20  "OMAPve_y_HMI_Popup_Status_2"
  OMAPve_y_TSR_Vision_Only_Sign_TypeNum/1 -> Bus Creator16/1  "OMAPve_y_TSR_Vision_Only_Sign_Type_2"
  OMAPve_y_TJA_status_iconNum/1 -> Bus Creator16/30  "OMAPve_y_TJA_status_icon_2"
  OMAPve_y_AEB_Fault_StatusNum/1 -> Bus Creator16/14  "OMAPve_y_AEB_Fault_Status_2"
  OMAPve_y_Vehicle_Lane_DisplayNum/1 -> Bus Creator16/21  "OMAPve_y_Vehicle_Lane_Display_2"
  OMAPve_y_LKA_Switch_StateNum/1 -> Bus Creator16/26  "OMAPve_y_LKA_Switch_State_2"
  OMAPve_y_LDW_FlagNum/1 -> Bus Creator16/22  "OMAPve_y_LDW_Flag_2"
  Bus Creator16/1 -> Default_IC/1  "Default_IC"
  OMAPve_y_ADAS_ELKStsNum1/1 -> Bus Creator16/28  "OMAPve_y_ADAS_ELKSts_2"
  Constant22/1 -> Bus Creator16/53  "OMAPve_y_ADAS_SRR-LF_ErrorSt"
  Constant20/1 -> Bus Creator16/51  "OMAPve_y_ADAS_SRR_LF_SystWorkSt"
  Constant26/1 -> Bus Creator16/57  "OMAPve_y_ADAS_SRR_RF_FCTAWrn"
  Constant10/1 -> Bus Creator16/41  "OMAPve_y_ADAS_BSD_RCTAWarning"
  Constant24/1 -> Bus Creator16/55  "OMAPve_y_ADAS_SRR_LF_FCTAWrn"
  Constant8/1 -> Bus Creator16/39  "OMAPve_y_ADAS_BSD_LCAWarning"
  Constant25/1 -> Bus Creator16/56  "OMAPve_y_ADAS_SRR_RF_SystStInfo"
  Constant9/1 -> Bus Creator16/40  "OMAPve_y_ADAS_BSD_DoorOpenWrn"
  Constant7/1 -> Bus Creator16/38  "OMAPve_y_ADAS_BSD_S_ErrorSt"
  Constant6/1 -> Bus Creator16/37  "OMAPve_y_ADAS_BSD_ErrorSt"
  Constant3/1 -> Bus Creator16/34  "OMAPve_y_ADAS_BSD_SystemStInfo"
  Constant2/1 -> Bus Creator16/33  "OMAPve_y_ADAS_SRR_SystemState"
  Constant5/1 -> Bus Creator16/36  "OMAPve_y_ADAS_BSD_S_LCWWorkSt"
  Constant12/1 -> Bus Creator16/43  "OMAPve_y_ADAS_BSD_S_DOWWorkSt"
  Constant11/1 -> Bus Creator16/42  "OMAPve_y_ADAS_BSD_DOWWorkingSt"
  Constant23/1 -> Bus Creator16/54  "OMAPve_y_ADAS_SRR-RF_ErrorSt"
  Constant21/1 -> Bus Creator16/52  "OMAPve_y_ADAS_SRR_RF_SystWorkSt"
  Constant18/1 -> Bus Creator16/49  "OMAPve_y_ADAS_BSD_S_RCTAWarning"
  Constant17/1 -> Bus Creator16/48  "OMAPve_y_ADAS_BSD_S_DoorOpenWrn"
  Constant/1 -> Bus Creator16/31  "OMAPve_y_ADAS_LeftLEDWarningSt"
  Constant19/1 -> Bus Creator16/50  "OMAPve_y_ADAS_SRR_LF_SystStInfo"
  Constant1/1 -> Bus Creator16/32  "OMAPve_y_ADAS_RighrLEDWarningSt"
  Constant13/1 -> Bus Creator16/44  "OMAPve_y_ADAS_BSD_RCTAWorkingSt"
  Constant16/1 -> Bus Creator16/47  "OMAPve_y_ADAS_BSD_S_LCAWarning"
  Constant15/1 -> Bus Creator16/46  "OMAPve_y_ADAS_BSD_S_SystStInfo"
  Constant4/1 -> Bus Creator16/35  "OMAPve_y_ADAS_BSD_LCWWorkingSt"
  Constant14/1 -> Bus Creator16/45  "OMAPve_y_ADAS_BSD_S_RCTAWorkSt"

== system OMAP_ver_MIL10/OMAP_Module/Default_OTHER ==
  Bus Creator26 : BusCreator  Inputs=5
  OMAPve_y_ABS_ESP_power_cut_request2Num : Constant  Value=0  OutDataTypeStr=uint8
  OMAPve_y_ASR_connection_dis_demand2Num : Constant  Value=0  OutDataTypeStr=uint8
  OMAPve_y_ECU_operating_phaseNum : Constant  Value=9  OutDataTypeStr=uint8
  OMAPve_y_Radar_StateNum : Constant  Value=2  OutDataTypeStr=uint8
  OMAPve_y_TYPE_RAPPORTNum : Constant  Value=0  OutDataTypeStr=uint8
  Default : Outport
  wires:
  OMAPve_y_ASR_connection_dis_demand2Num/1 -> Bus Creator26/2  "OMAPve_y_ASR_connection_dis_demand2_2"
  OMAPve_y_ABS_ESP_power_cut_request2Num/1 -> Bus Creator26/1  "OMAPve_y_ABS_ESP_power_cut_request2_2"
  OMAPve_y_TYPE_RAPPORTNum/1 -> Bus Creator26/3  "OMAPve_y_TYPE_RAPPORT_2"
  Bus Creator26/1 -> Default/1  "Default"
  OMAPve_y_Radar_StateNum/1 -> Bus Creator26/5  "OMAPve_y_Radar_State_2"
  OMAPve_y_ECU_operating_phaseNum/1 -> Bus Creator26/4  "OMAPve_y_ECU_operating_phase_2"
